simulink model "exampleCAM"  (R2020a)
settings: Solver=FixedStepDiscrete  StartTime=0.0  StopTime=inf  RelTol=1e-3
libraries: aerolibanimutils x1, visionsinks x1
settings Model: Creator=i72GBSentey  LastModifiedBy=Desktop-dds

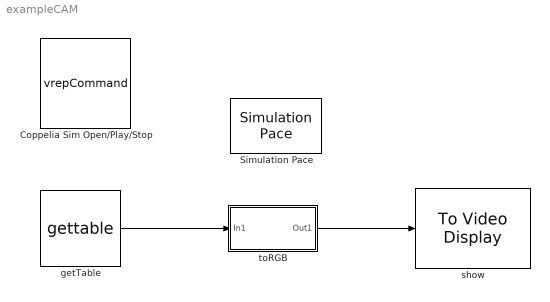
== system exampleCAM ==
  Coppelia Sim Open/Play/Stop : S-Function  FunctionName=vrepCommand  Parameters=scene  SFunctionDeploymentMode=off  EnableBusSupport=off  mask{scene='exampleCAM.ttt'}
      mask prompts: scene "V-rep Scene Name"
      mask Display: image('play_stop.png')
  Simulation Pace : aerolibanimutils/Simulation Pace  SimulationPace=1  SleepMode=Auto  OutputPaceError=off  SampleTime=1/30
  getTable : S-Function  FunctionName=gettable  Parameters=tname  SFunctionDeploymentMode=off  EnableBusSupport=off  mask{tname='VREPCAM'}
      mask prompts: tname "Table Name"
      mask DialogControl DescGroupVar Prompt: GetData
      mask DialogControl DescTextVar Prompt: Gets the data from a table declared in CoppeliaSim
      mask Display: image("CoppeliaSim.png")
  show : visionsinks/To Video Display  windowSizeMode=Normal  openAtMdlStart=on  fullScreen=off  videoWindowX=1  videoWindowY=31  saveWindowSize=off  videoWindowWidth=718  videoWindowHeight=828  inputColorFormat=RGB  inputType=Obsolete  imagePorts=One multidimensional signal  OutputDevice=On-screen video monitor  dataOrg=Column-major  isWindowOpen=off
  "toRGB " : Subsystem  mask{ResX=512, ResY=512}
      mask prompts: ResX "Resolucion Camara X"; ResY "Resolucion Camara Y"
      mask Display:
      | port_label('output', 1, 'RGB')
      | port_label('input', 1, 'videoIN')
  wires:
  getTable/1 -> "toRGB "/1(In1)
  "toRGB "/1(Out1) -> show/1

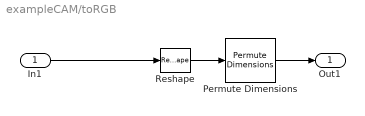
== system exampleCAM/toRGB  ==
  In1 : Inport  OutDataTypeStr=uint8  PortDimensions=512*512*3
  Permute Dimensions : PermuteDimensions  Order=[3 2 1]
  Reshape : Reshape  OutputDimensionality=Customize  OutputDimensions=[3,ResX,ResY]
  Out1 : Outport  VectorParamsAs1DForOutWhenUnconnected=off
  wires:
  Permute Dimensions/1 -> Out1/1
  Reshape/1 -> Permute Dimensions/1
  In1/1 -> Reshape/1
